simulink library "INT_BattU_DD"  (R2016b)
settings: Solver=VariableStepAuto  StartTime=0.0  StopTime=10.0  RelTol=1e-3
settings Model: Creator=Administrator  LastModifiedBy=Administrator

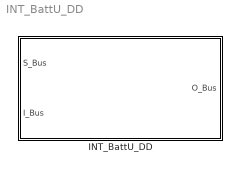
== system INT_BattU_DD ==
  INT_BattU_DD : Subsystem

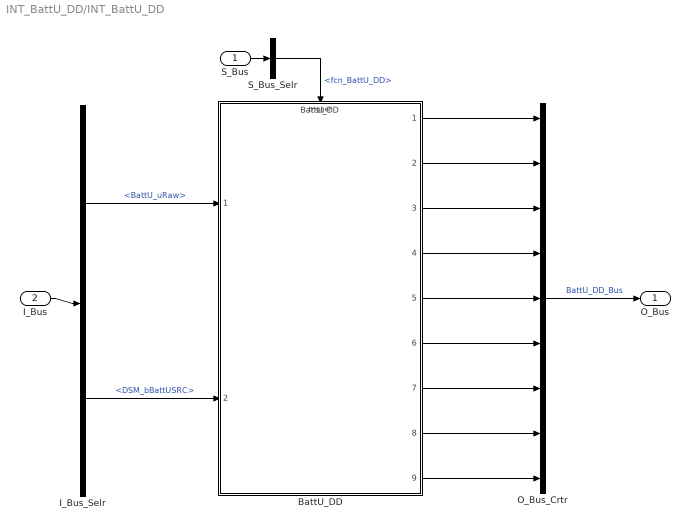
== system INT_BattU_DD/INT_BattU_DD ==
  S_Bus : Inport
  I_Bus : Inport  Port=2
  BattU_DD : ModelReference  ModelNameDialog=BattU_DD  SimulationMode=Normal  ModelReferenceVersion=1.8  TriggerPortName=function  TriggerPortTriggerType=function-call  TriggerPortStatesWhenEnabling=held
  I_Bus_Selr : BusSelector  OutputSignals=BattU_uRaw,DSM_bBattUSRC
  O_Bus_Crtr : BusCreator  Inputs=9
  S_Bus_Selr : BusSelector  OutputSignals=fcn_BattU_DD
  O_Bus : Outport
  wires:
  S_Bus_Selr/1 -> BattU_DD/Trigger  "<fcn_BattU_DD>"
  S_Bus/1 -> S_Bus_Selr/1
  I_Bus/1 -> I_Bus_Selr/1
  I_Bus_Selr/1 -> BattU_DD/1  "<BattU_uRaw>"
  I_Bus_Selr/2 -> BattU_DD/2  "<DSM_bBattUSRC>"
  O_Bus_Crtr/1 -> O_Bus/1  "BattU_DD_Bus"
  BattU_DD/1 -> O_Bus_Crtr/1
  BattU_DD/2 -> O_Bus_Crtr/2
  BattU_DD/3 -> O_Bus_Crtr/3
  BattU_DD/4 -> O_Bus_Crtr/4
  BattU_DD/5 -> O_Bus_Crtr/5
  BattU_DD/6 -> O_Bus_Crtr/6
  BattU_DD/7 -> O_Bus_Crtr/7
  BattU_DD/8 -> O_Bus_Crtr/8
  BattU_DD/9 -> O_Bus_Crtr/9
